simulink model "workshop_boat_blank"  (R2022b)
settings: Solver=ode15s  StartTime=0.0  StopTime=45  RelTol=1e-6  AbsTol=1e-6  EnableMultiTasking=on
undefined symbols (not defined in the file or in its folder): disk, sigbuilder_block, X, Y, Z
libraries: sm_lib x4, nesl_utility x2
settings Model: Creator=bhorton  LastModifiedBy=rlachaux
settings SolverCC: ZeroCrossAlgorithm=Adaptive  AlgebraicLoopSolver=TrustRegion
settings DataIOCC: LimitDataPoints=on  MaxDataPoints=10000
settings OptimizationCC: LifeSpan=inf
settings DebuggingCC: UnconnectedInputMsg=warning  UnconnectedOutputMsg=warning  UnconnectedLineMsg=warning  AllowSymbolicDim=off  SFUnexpectedBacktrackingDiag=warning  SFNoUnconditionalDefaultTransitionDiag=warning  SFExecutionAtInitializationDiag=none  SFMachineParentedDataDiag=warning  ArithmeticOperatorsInVariantConditions=warning
settings ModelReferenceCC: EnableRefExpFcnMdlSchedulingChecks=on
settings SFSimCC: SimUseLocalCustomCode=off  CustomCodeUndefinedFunction=UseInterfaceOnly
settings RTWCC: RTWUseLocalCustomCode=off  DLArmComputeVersion=19.05
settings CodeAppCC: StateflowObjectComments=on
settings GRTTargetCC: TargetLangStandard=C89/C90 (ANSI)
settings ConfigComp: CovMetricSettings=dw  CovSaveCumulativeToWorkspaceVar=on  CovSaveSingleToWorkspaceVar=on  CovExternalEMLEnable=off  CovSFcnEnable=off
settings SimscapeCC: SimscapeLogType=all  SimscapeLogSimulationStatistics=on  SimscapeLogDataHistory=10000
settings ExplorerConfigSet: InternalSimMechanicsExplorerSettings="<ExplorerConfiguration><canonicalview>default</canonicalview><AnimationSetting><BasePlaybackSpeed>1.0</BasePlaybackSpeed><PlaybackSpeedFactor>1.0</PlaybackSpeedFactor></AnimationSetting><TilePanel><TileInfo><Tiles Columns=\"2\" Count=\"3\" Rows=\"2\"><Column Weight=\"0.5\"/><Column Weight=\"0.5\"/><Row Weight=\"0.4994\"/><Row Weight=\"0.5006\"/><Tile Height=\"2\" Width=\"1\" X=\"0\" Y=\"0\"/><Tile Height=\"1\" Width=\"1\" X=\"1\" Y=\"0\"/><Tile Height=\"1\" Width=\"1\" X=\"1\" Y=\"1\"/></Tiles></TileInfo><SceneInfo><SceneViewer><BGColor><R>0.60000002384185791</R><G>0.60000002384185791</G><B>0.60000002384185791</B></BGColor><Camera><DoPerspective>off</DoPerspective><Position><X>2.72907980115163751</X><Y>1.63827710737355892</Y><Z>5.84466597133086818</Z></Position><Center><X>1.48957165804863778</X><Y>-0.312477395456248752</Y><Z>2.71114995707715156</Z></Center><Up><X>0.0871556787867786148</X><Y>0.8298702872998307</Y><Z>-0.551107243567087735</Z></Up><ViewLimDist>1</ViewLimDist><YLim>5.28419304463390116</YLim><XLim>3.96508464876347055</XLim></Camera></SceneViewer><SceneViewer><BGColor><R>0.60000002384185791</R><G>0.60000002384185791</G><B>0.60000002384185791</B></BGColor><Camera><DoPerspective>off</DoPerspective><Position><X>0.174100554176560618</X><Y>2.79843990503689621</Y><Z>0.284823193336330216</Z></Position><Center><X>0.177652103694306729</X><Y>-0.924710698878394188</Y><Z>0.283383219246318929</Z></Center><Up><X>0.00583965905908712894</X><Y>0.000392326129121878253</Y><Z>-0.999982872084458463</Z></Up><ViewLimDist>1</ViewLimDist><YLim>0.869664947050413972</YLim><XLim>1.32261544030583789</XLim></Camera></SceneViewer><SceneViewer><BGColor><R>0.60000002384185791</R><G>0.60000002384185791</G><B>0.60000002384185791</B></BGColor><Camera><DoPerspective>off</DoPerspective><Position><X>-0.273643330341835023</X><Y>-1.00050075945724948</Y><Z>3.47750989252231513</Z></Position><Center><X>-0.273643330341835023</X><Y>-1.00050075945724948</Y><Z>-3.69061607941034708e-08</Z></Center><Up><X>0</X><Y>1</Y><Z>-0</Z></Up><ViewLimDist>1</ViewLimDist><YLim>2.77031267511226043</YLim><XLim>4.21318386006656276</XLim></Camera></SceneViewer></SceneInfo></TilePanel><MechEditorPanel><Cameras/><GfxPanelCameraMap/><VideoCreator><PlaybackSpeedRatio>1.0</PlaybackSpeedRatio><FrameRate>30</FrameRate><VideoFormat>Motion JPEG AVI</VideoFormat><FrameSize>auto</FrameSize></VideoCreator></MechEditorPanel></ExplorerConfiguration>"

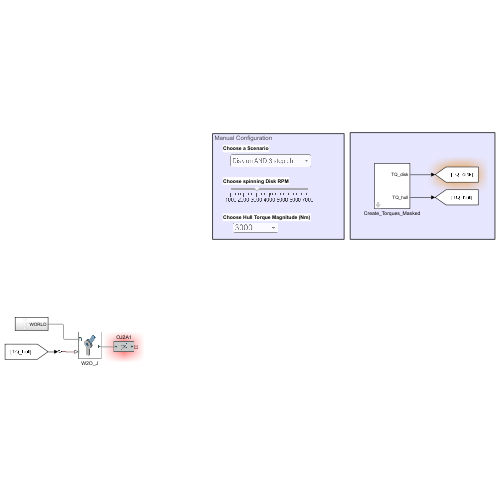
[thumbnail: Simulink's stored preview of the top-level diagram]
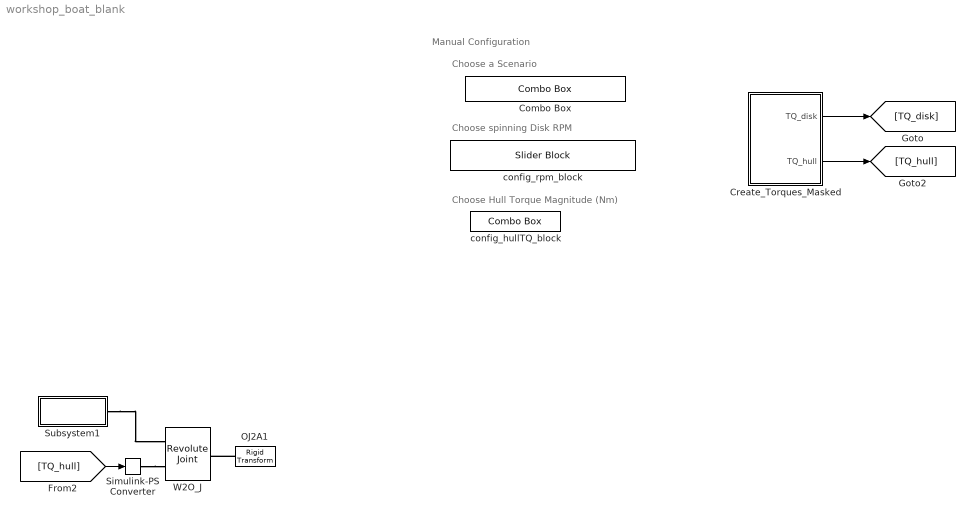
== system workshop_boat_blank ==
  note: Choose a Scenario
  note: Manual Configuration
  note: Choose spinning Disk RPM
  note: Choose Hull Torque Magnitude (Nm)
  Combo Box : ComboBox  LabelPosition=Hide  SelectedLabel=Disk on AND 3 step changes
      settings: Values={{'NO Stabilization (disk is NOT spinning)', 'Spin up disk BEFORE Disturbance', 'Spin up disk AFTER disturbance', 'Disk always spinning', 'Disk on AND 3 step changes', 'Spin Ramp to 10 percent'}, [1 2 3 4 5 6]}
  Create_Torques_Masked : Subsystem  mask{the_scenario=5, the_disk_rpm=3025.477707006369, the_tau_hull=3000}
      mask prompts: the_scenario "Scenario ID"; the_disk_rpm "Disk RPM"; the_tau_hull "Magnitude of HULL torque (N.m)"
      mask init:
      | THE_BLOCK = [gcb,'/my_sig_builder'];
      | signalbuilder(THE_BLOCK,'activegroup',the_scenario)
  OJ2A1 : sm_lib/Frames and Transforms/Rigid Transform  TranslationMethod=Cartesian  TranslationStandardOffset=0  TranslationLengthUnit=m  TranslationStandardAxis=+Z  TranslationCartesianOffset=my_points.A_rel2O  TranslationROffset=0  TranslationROffsetUnits=m  TranslationZOffset=0  TranslationZOffsetUnits=m  TranslationThetaOffset=0  TranslationThetaOffsetUnits=deg  RotationMethod=None  RotationAngleUnits=deg  RotationStandardAxis=+Z  RotationAngle=0.0  RotationArbitraryAxis=[0 0 1]  FollAlignAxisA=+Z  BaseAlignAxisA=+Y  FollAlignAxisB=+X  BaseAlignAxisB=+X  RotationSequenceAxes=FollowerAxes  RotationSequence=XYX  RotationSequenceAngles=[0 0 0]  RotationSequenceAnglesUnits=deg  RotationMatrix=[1 0 0; 0 1 0; 0 0 1]  Quaternion=[1 0 0 0]
  Simulink-PS Converter : nesl_utility/Simulink-PS Converter  PhysicalDomain=network_engine_domain  SubClassName=ps_input  LeftPortType=input  RightPortType=output  PseudoPeriodic=off  Frequencies=[]  NoiseDistribution=none  NoiseParameters=[]  Unit=1  AffineConversion=off  FilteringAndDerivatives=provide  SimscapeFilterOrder=1  InputFilterTimeConstant=0.001  UdotUserProvided=0
  Subsystem1 : Subsystem
  W2O_J : sm_lib/Joints/Revolute Joint  JointMode=Normal  SenseConstraintForce=off  SenseConstraintForceX=off  SenseConstraintForceY=off  SenseConstraintForceZ=off  SenseConstraintTorque=off  SenseConstraintTorqueX=off  SenseConstraintTorqueY=off  SenseConstraintTorqueZ=off  SenseTotalForce=off  SenseTotalForceX=off  SenseTotalForceY=off  SenseTotalForceZ=off  SenseTotalTorque=off  SenseTotalTorqueX=off  SenseTotalTorqueY=off  SenseTotalTorqueZ=off  CompositeWrenchDir=FollowerOnBase  CompositeWrenchFrame=BaseFrame  EquilibriumPosition=0  EquilibriumPositionUnits=deg  SpringStiffness=0  SpringStiffnessUnits=N*m/deg  DampingCoefficient=0  DampingCoefficientUnits=N*m/(deg/s)  TorqueActuationMode=InputTorque  MotionActuationMode=ComputedMotion  SensePosition=off  SenseVelocity=off  SenseAcceleration=off  SenseTorqueForce=off  SenseLowerLimitTorqueForce=off  SenseUpperLimitTorqueForce=off  LowerLimitSpecify=off  LowerLimitBound=-90  LowerLimitBoundUnits=deg  LowerLimitStiffness=1e4  LowerLimitStiffnessUnits=N*m/deg  LowerLimitDamping=10  LowerLimitDampingUnits=N*m/(deg/s)  LowerLimitTransitionRegionWidth=0.1  LowerLimitTransitionRegionWidthUnits=deg  UpperLimitSpecify=off  UpperLimitBound=90  UpperLimitBoundUnits=deg  UpperLimitStiffness=1e4  UpperLimitStiffnessUnits=N*m/deg  UpperLimitDamping=10  UpperLimitDampingUnits=N*m/(deg/s)  UpperLimitTransitionRegionWidth=0.1  UpperLimitTransitionRegionWidthUnits=deg  PositionTargetSpecify=off  PositionTargetPriority=High  PositionTargetValue=0  PositionTargetValueUnits=deg  VelocityTargetSpecify=off  VelocityTargetPriority=High  VelocityTargetValue=0  VelocityTargetValueUnits=deg/s
  config_hullTQ_block : ComboBox  LabelPosition=Hide  SelectedLabel=3000
      settings: Values={{'1000', '3000', '5000', '7000', '9000', '11000'}, [1000 3000 5000 7000 9000 11000]}
  config_rpm_block : SliderBlock  LabelPosition=Hide  ScaleMin=1000  ScaleMax=7000  TickInterval=1000
  wires:
  [TQ_hull] -> Simulink-PS Converter/1
  Create_Torques_Masked/1(TQ_disk) -> [TQ_disk]
  Create_Torques_Masked/2(TQ_hull) -> [TQ_hull]
  connections:
  Subsystem1/RConn1 -- W2O_J/LConn1
  OJ2A1/LConn1 -- W2O_J/RConn1
  Simulink-PS Converter/RConn1 -- W2O_J/LConn2

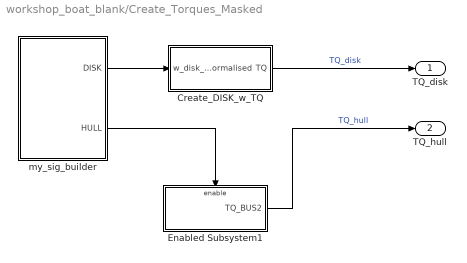
== system workshop_boat_blank/Create_Torques_Masked ==
  Create_DISK_w_TQ : Subsystem
  Enabled Subsystem1 : Subsystem  TreatAsAtomicUnit=on
  my_sig_builder : Subsystem  Tag=STV Subsys  LoadFcn=sigbuilder_block('load');  StartFcn=sigbuilder_block('start');  StopFcn=sigbuilder_block('stop');  ClipboardFcn=sigbuilder_block('clipboard');  mask(Sigbuilder block){tuvar=[0:10]}
      mask help: Simulink:masks:SigbuilderBlock_MD
      mask init:
      | if ~strcmp(get_param(bdroot(gcbh),'SimulationStatus'),'stopped') tuvar = sigbuilder_block('maskInit'); end
      settings: CopyFcn=sigbuilder_block('copy');  DeleteFcn=sigbuilder_block('delete');  ModelCloseFcn=sigbuilder_block('modelClose');  PreSaveFcn=sigbuilder_block('preSave');  PauseFcn=sigbuilder_block('pause');  ContinueFcn=sigbuilder_block('continue');  NameChangeFcn=sigbuilder_block('namechange');  OpenFcn=sigbuilder_block('open',[437.6 199.2 550.4 400 ]);  CloseFcn=sigbuilder_block('close');
      mask Display: plot(0, 0, 100, 100,[2, 2, 32, 32, 2], [68, 8, 8, 68, 68],[32, 2], [38, 38], [32, 19, 2],[53, 60, 44], [32, 17, 17, 2],[16, 16, 31, 31]);txt = getActiveGroup(gcbh);text(2, 100, txt,'verticalAlignment', 'top');
  TQ_disk : Outport
  TQ_hull : Outport  Port=2
  wires:
  my_sig_builder/1(DISK) -> Create_DISK_w_TQ/1(w_disk_normalised)
  Create_DISK_w_TQ/1(TQ) -> TQ_disk/1  "TQ_disk"
  Enabled Subsystem1/1(TQ_BUS2) -> TQ_hull/1  "TQ_hull"
  my_sig_builder/2(HULL) -> Enabled Subsystem1/Enable

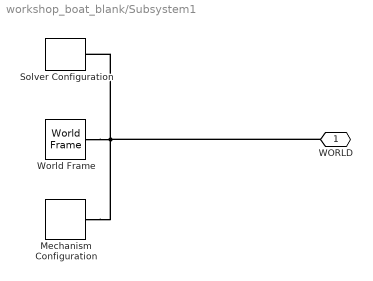
== system workshop_boat_blank/Subsystem1 ==
  Mechanism Configuration : sm_lib/Utilities/Mechanism Configuration  UniformGravity=Constant  GravityVector=[0 -9.80665 0]  GravityUnits=m/s^2  LinearizationDelta=0.001  JointModeTransitionNonlinearIterations=2
  Solver Configuration : nesl_utility/Solver Configuration  PhysicalDomain=network_engine_domain  SubClassName=solver  LeftPortType=input  RightPortType=generic  Tones=[]  Harmonics=[]  SimulateNoise=off  Profile=off  UseLocalSampling=off  EnableSwitchedLinearOptims=on  FrequencyDomain=off  UseCCode=off  RelTol=0.001  AbsTol=1e-06  MinStep=1e-09  ToWorkspace=off  RevertToSquareIcSolve=off  NumHomotopyIterations=100  PhasorMode=off  PhasorModeNumHarmonics=1  ConsistencySolver=NEWTON_FTOL  IndexReductionMethod=DerivativeReplacement  DoDC=off  ResidualTolerance=1e-09  ConsistencyTolSource=GLOBAL  ConsistencyAbsTol=0.001  ConsistencyRelTol=0.001  ConsistencyTolFactor=0.001  UseLocalSolver=off  LocalSolverChoice=NE_BACKWARD_EULER_ADVANCER  ResolveIndetEquations=on  FunctionEvalNumThread=1  LocalSolverSampleTime=0.001  DoFixedCost=off  MaxNonlinIter=3  MaxModeIter=2  ComputeImpulses=off  ImpulseIterations=2  LinearAlgebra=Sparse  LinearAlgebraNumThread=0  EquationFormulation=NE_TIME_EF  DelaysMemoryBudget=1024  AutomaticFiltering=on  FilteringTimeConstant=0.001  PartitionStorageMethod=AS_NEEDED  PartitionMemoryBudget=1024  PartitionMethod=FAST
  World Frame : sm_lib/Frames and Transforms/World Frame
  WORLD : PMIOPort  Side=Right
  connections:
  World Frame/RConn1 -- Mechanism Configuration/RConn1 -- WORLD/RConn1 -- Solver Configuration/RConn1

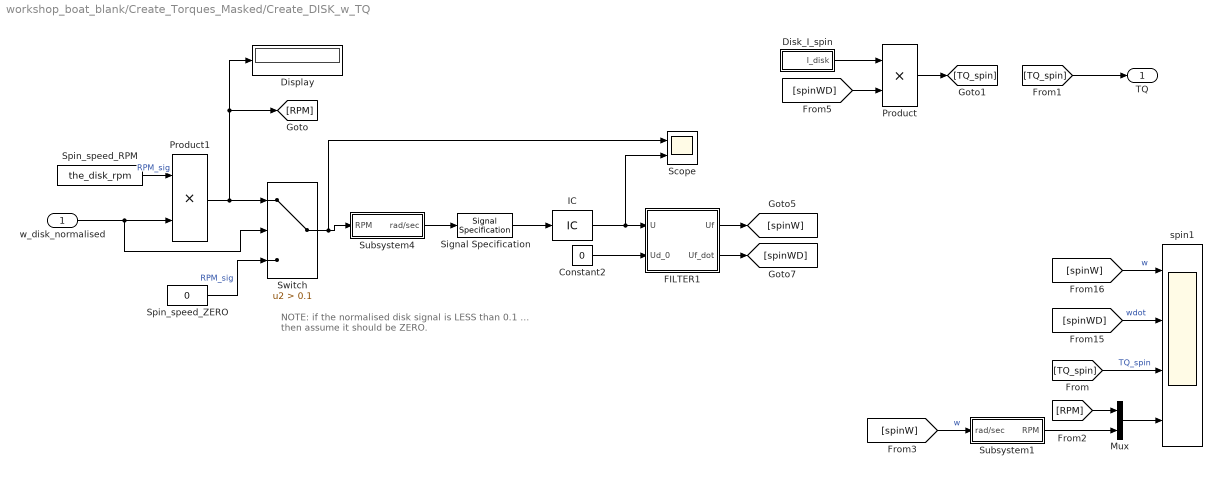
== system workshop_boat_blank/Create_Torques_Masked/Create_DISK_w_TQ ==
  note: NOTE:  if the normalised disk signal
      | is LESS than 0.1 ... then assume it should be ZERO.
  w_disk_normalised : Inport
  Constant2 : Constant  Value=0
  Disk_I_spin : Subsystem
  Display : Display
  FILTER1 : Subsystem
  IC : InitialCondition  Value=0
  Mux : Mux  Inputs=2
  Product : Product
  Product1 : Product
  Scope : Scope  NumInputPorts=2
  Signal Specification : SignalSpecification  SampleTime=0
  Spin_speed_RPM : Constant  Value=the_disk_rpm
  Spin_speed_ZERO : Constant  Value=0
  Subsystem1 : Subsystem
  Subsystem4 : Subsystem
  Switch : Switch  Criteria=u2 > Threshold  Threshold=0.1  SaturateOnIntegerOverflow=off  InputSameDT=off
  spin1 : Scope  NumInputPorts=4
  TQ : Outport
  wires:
  [spinW] -> spin1/1  "w"
  Product/1 -> [TQ_spin]
  Disk_I_spin/1(I_disk) -> Product/1
  [spinWD] -> Product/2
  [spinWD] -> spin1/2  "wdot"
  Constant2/1 -> FILTER1/2(Ud_0)
  FILTER1/1(Uf) -> [spinW]
  FILTER1/2(Uf_dot) -> [spinWD]
  Switch/1 -> Scope/1, Subsystem4/1(RPM)
  [TQ_spin] -> spin1/3  "TQ_spin"
  [TQ_spin] -> TQ/1
  Spin_speed_ZERO/1 -> Switch/3  "RPM_sig"
  IC/1 -> Scope/2, FILTER1/1(U)
  Subsystem4/1(rad/sec) -> Signal Specification/1
  Signal Specification/1 -> IC/1
  Mux/1 -> spin1/4
  [RPM] -> Mux/1
  [spinW] -> Subsystem1/1(rad/sec)  "w"
  Subsystem1/1(RPM) -> Mux/2
  w_disk_normalised/1 -> Switch/2, Product1/2
  Spin_speed_RPM/1 -> Product1/1  "RPM_sig"
  Product1/1 -> Switch/1, [RPM], Display/1

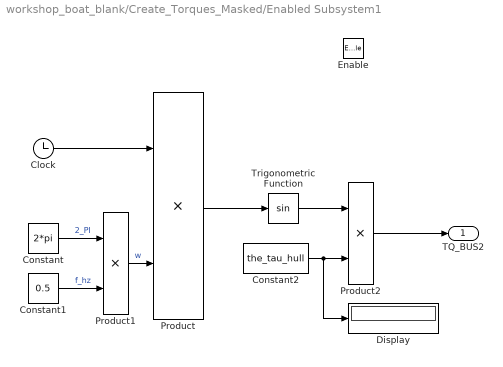
== system workshop_boat_blank/Create_Torques_Masked/Enabled Subsystem1 ==
  Enable : EnablePort  StatesWhenEnabling=reset
  Clock : Clock
  Constant : Constant  Value=2*pi
  Constant1 : Constant  Value=0.5
  Constant2 : Constant  Value=the_tau_hull
  Display : Display
  Product : Product
  Product1 : Product
  Product2 : Product
  Trigonometric Function : Trigonometry
  TQ_BUS2 : Outport  InitialOutput=0
  wires:
  Product/1 -> Trigonometric Function/1
  Constant1/1 -> Product1/2  "f_hz"
  Product2/1 -> TQ_BUS2/1
  Constant/1 -> Product1/1  "2_PI"
  Clock/1 -> Product/1
  Product1/1 -> Product/2  "w"
  Trigonometric Function/1 -> Product2/1
  Constant2/1 -> Display/1, Product2/2

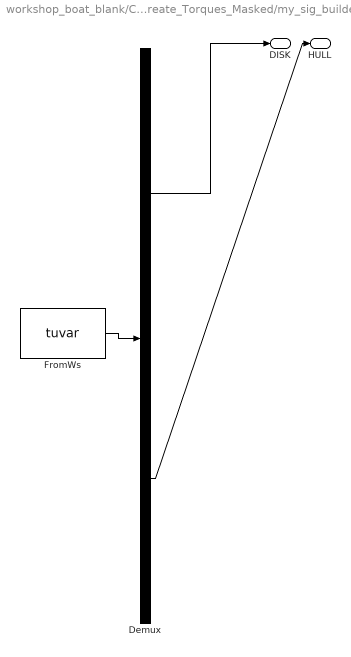
== system workshop_boat_blank/Create_Torques_Masked/my_sig_builder ==
  Demux : Demux  Tag=STV Demux  Outputs=2
      settings: DisplayOption=none
  FromWs : FromWorkspace  Tag=STV FromWs  VariableName=tuvar
      SigBuilderData=|
      | common.afterFinalStr = 'Extrapolate'
      | common.sampleTime = 0
      | dataSet(1).timeRange = [0 60]
      | dataSet(1).name = 'NO_STABILIZATION'
      | dataSet(2).timeRange = [0 60]
      | dataSet(2).name = 'DISK_THEN_LOAD'
      | dataSet(3).timeRange = [0 60]
      | dataSet(3).name = 'LOAD_THEN_DISK'
      | dataSet(4).timeRange = [0 60]
      | dataSet(4).name = 'DISK_THEN_LOAD_V2'
      | dataSet(5).timeRange = [0 60]
      | dataSet(5).name = 'DISK_ON_AND_3_STEP_CHANGES'
      | dataSet(6).timeRange = [0 60]
      | dataSet(6).name = 'RAMP_TO_10PC'
      | sbobj.Groups(1).Name = 'NO_STABILIZATION'
      | sbobj.Groups(1).Signals(1).Name = 'DISK'
      | sbobj.Groups(1).Signals(1).XData = [0 60]
      | sbobj.Groups(1).Signals(1).YData = [0 0]
      | sbobj.Groups(1).Signals(2).Name = 'HULL'
      | sbobj.Groups(1).Signals(2).XData = [0 10.2 10.2 36 60]
      | sbobj.Groups(1).Signals(2).YData = [0 0 1 1 1]
      | sbobj.Groups(1).TimeRange = [0 60]
      | sbobj.Groups(2).Name = 'DISK_THEN_LOAD'
      | sbobj.Groups(2).Signals(1).Name = 'DISK'
      | sbobj.Groups(2).Signals(1).XData = [0 5 29.99 30 60]
      | sbobj.Groups(2).Signals(1).YData = [1 1 1 0 0]
      | sbobj.Groups(2).Signals(2).Name = 'HULL'
      | sbobj.Groups(2).Signals(2).XData = [0 10.2 10.2 36 60]
      | sbobj.Groups(2).Signals(2).YData = [0 0 1 1 1]
      | sbobj.Groups(2).TimeRange = [0 60]
      | sbobj.Groups(3).Name = 'LOAD_THEN_DISK'
      | sbobj.Groups(3).Signals(1).Name = 'DISK'
      | sbobj.Groups(3).Signals(1).XData = [0 10 10 30 30 60]
      | sbobj.Groups(3).Signals(1).YData = [0 0 1 1 0 0]
      | sbobj.Groups(3).Signals(2).Name = 'HULL'
      | sbobj.Groups(3).Signals(2).XData = [0 10.2 36 60]
      | sbobj.Groups(3).Signals(2).YData = [1 1 1 1]
      | sbobj.Groups(3).TimeRange = [0 60]
      | sbobj.Groups(4).Name = 'DISK_THEN_LOAD_V2'
      | sbobj.Groups(4).Signals(1).Name = 'DISK'
      | sbobj.Groups(4).Signals(1).XData = [0 5 20 60]
      | sbobj.Groups(4).Signals(1).YData = [1 1 1 1]
      | sbobj.Groups(4).Signals(2).Name = 'HULL'
      | sbobj.Groups(4).Signals(2).XData = [0 10.2 10.2 36 60]
      | sbobj.Groups(4).Signals(2).YData = [0 0 1 1 1]
      | sbobj.Groups(4).TimeRange = [0 60]
      | sbobj.Groups(5).Name = 'DISK_ON_AND_3_STEP_CHANGES'
      | sbobj.Groups(5).Signals(1).Name = 'DISK'
      | sbobj.Groups(5).Signals(1).XData = [0 5 20 20 30 30 40 40 60]
      | sbobj.Groups(5).Signals(1).YData = [1 1 1 0.7 0.7 0.4 0.4 1 1]
      | sbobj.Groups(5).Signals(2).Name = 'HULL'
      | sbobj.Groups(5).Signals(2).XData = [0 10.2 10.2 36 60]
      | sbobj.Groups(5).Signals(2).YData = [0 0 1 1 1]
      | sbobj.Groups(5).TimeRange = [0 60]
      | sbobj.Groups(6).Name = 'RAMP_TO_10PC'
      | sbobj.Groups(6).Signals(1).Name = 'DISK'
      | sbobj.Groups(6).Signals(1).XData = [0 60]
      | sbobj.Groups(6).Signals(1).YData = [1 0.1]
      | sbobj.Groups(6).Signals(2).Name = 'HULL'
      | sbobj.Groups(6).Signals(2).XData = [0 10.2 10.2 36 60]
      | sbobj.Groups(6).Signals(2).YData = [0 0 1 1 1]
      | sbobj.Groups(6).TimeRange = [0 60]
  DISK : Outport  Tag=STV Outport
  HULL : Outport  Tag=STV Outport  Port=2
  wires:
  FromWs/1 -> Demux/1
  Demux/1 -> DISK/1
  Demux/2 -> HULL/1

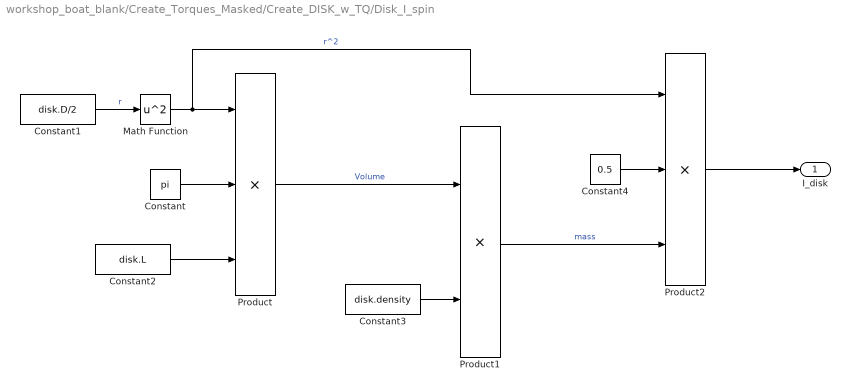
== system workshop_boat_blank/Create_Torques_Masked/Create_DISK_w_TQ/Disk_I_spin ==
  Constant : Constant  Value=pi
  Constant1 : Constant  Value=disk.D/2
  Constant2 : Constant  Value=disk.L
  Constant3 : Constant  Value=disk.density
  Constant4 : Constant  Value=0.5
  Math Function : Math  Operator=square
  Product : Product  Inputs=3
  Product1 : Product
  Product2 : Product  Inputs=3
  I_disk : Outport
  wires:
  Constant1/1 -> Math Function/1  "r"
  Math Function/1 -> Product2/1, Product/1  "r^2"
  Constant/1 -> Product/2
  Constant2/1 -> Product/3
  Constant3/1 -> Product1/2
  Product/1 -> Product1/1  "Volume"
  Product1/1 -> Product2/3  "mass"
  Constant4/1 -> Product2/2
  Product2/1 -> I_disk/1

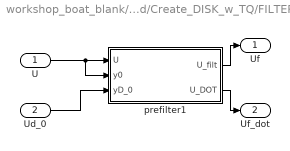
== system workshop_boat_blank/Create_Torques_Masked/Create_DISK_w_TQ/FILTER1 ==
  U : Inport
  Ud_0 : Inport  Port=2
  prefilter1 : Subsystem  mask(Derivative Estimation){wn=2*pi*5/5, p=1}
      mask prompts: wn "Natural frequency, wn (rad/sec)"; p "Damping ratio, p"
      mask help:
      | A simple derivative estimator using a 2nd order representation between input and output.
      |
      | The integrators use a discrete FORWARd Euler rule, and a sample time needs to be specified.
      mask init:
      | str1 = sprintf('wn = %.2f', wn);
      | str2 = sprintf('p  = %.2f', p);
      | %str3 = sprintf('dt = %.2f', dt);
      | %str = char(str1,str2,str3);
      | %str3 = sprintf('dt = %.2f', dt);
      | str = char(str1,str2);
      mask Display: disp(str)
  Uf : Outport  VectorParamsAs1DForOutWhenUnconnected=off
  Uf_dot : Outport  Port=2  VectorParamsAs1DForOutWhenUnconnected=off
  wires:
  Ud_0/1 -> prefilter1/3(yD_0)
  prefilter1/2(U_DOT) -> Uf_dot/1
  prefilter1/1(U_filt) -> Uf/1
  U/1 -> prefilter1/2(y0), prefilter1/1(U)

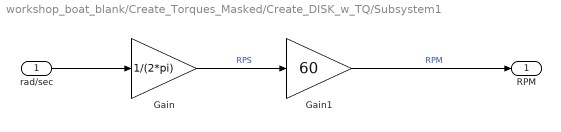
== system workshop_boat_blank/Create_Torques_Masked/Create_DISK_w_TQ/Subsystem1 ==
  rad/sec : Inport
  Gain : Gain  Gain=1/(2*pi)
  Gain1 : Gain  Gain=60
  RPM : Outport  VectorParamsAs1DForOutWhenUnconnected=off
  wires:
  rad/sec/1 -> Gain/1
  Gain/1 -> Gain1/1  "RPS"
  Gain1/1 -> RPM/1  "RPM"

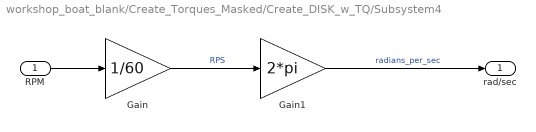
== system workshop_boat_blank/Create_Torques_Masked/Create_DISK_w_TQ/Subsystem4 ==
  RPM : Inport
  Gain : Gain  Gain=1/60
  Gain1 : Gain  Gain=2*pi
  rad/sec : Outport  VectorParamsAs1DForOutWhenUnconnected=off
  wires:
  RPM/1 -> Gain/1
  Gain/1 -> Gain1/1  "RPS"
  Gain1/1 -> rad/sec/1  "radians_per_sec"

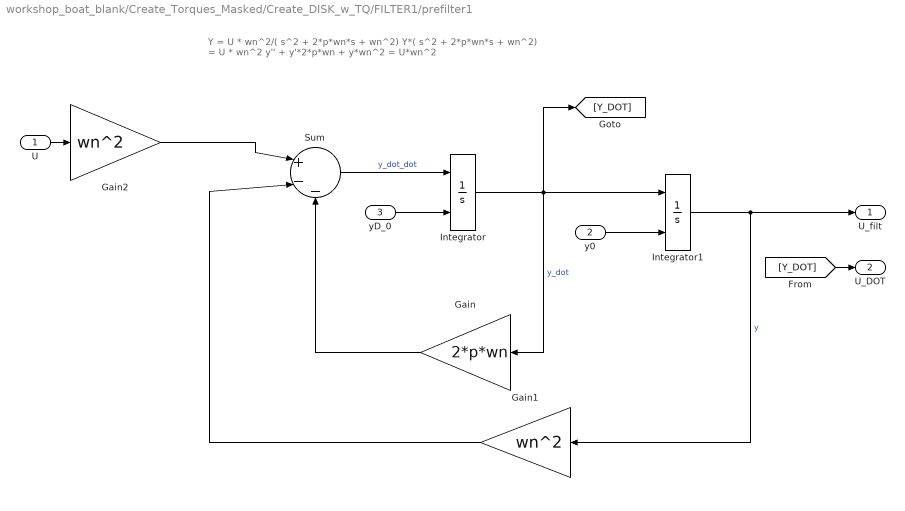
== system workshop_boat_blank/Create_Torques_Masked/Create_DISK_w_TQ/FILTER1/prefilter1 ==
  note: Y = U *     wn^2/( s^2 + 2*p*wn*s + wn^2)
      | Y*( s^2 + 2*p*wn*s + wn^2) = U * wn^2
      |
      | y'' + y'*2*p*wn + y*wn^2 = U*wn^2
  U : Inport
  y0 : Inport  Port=2
  yD_0 : Inport  Port=3
  Gain : Gain  Gain=2*p*wn
  Gain1 : Gain  Gain=wn^2
  Gain2 : Gain  Gain=wn^2
  Integrator : Integrator  InitialConditionSource=external
  Integrator1 : Integrator  InitialConditionSource=external
  Sum : Sum  Inputs=|+--
  U_filt : Outport  VectorParamsAs1DForOutWhenUnconnected=off
  U_DOT : Outport  Port=2  VectorParamsAs1DForOutWhenUnconnected=off
  wires:
  Integrator/1 -> [Y_DOT], Gain/1, Integrator1/1  "y_dot"
  Sum/1 -> Integrator/1  "y_dot_dot"
  Integrator1/1 -> Gain1/1, U_filt/1  "y"
  U/1 -> Gain2/1
  Gain2/1 -> Sum/1
  Gain/1 -> Sum/3
  Gain1/1 -> Sum/2
  [Y_DOT] -> U_DOT/1
  yD_0/1 -> Integrator/2
  y0/1 -> Integrator1/2
